simulink model "pid_extended_state_observor_pendulum"  (R2019b)
settings: Solver=FixedStepAuto  StartTime=0.0  StopTime=20  FixedStep=0.001  RelTol=1e-3
values from neighbouring files (symbols this model uses):
  L = [3*wd 3*wd^2 wd^3]'    [eso_design.m]
  wn = 1    [eso_design.m]
  zeta = 0.1    [eso_design.m]
libraries: simulink x1
settings Model: Creator=henry  LastModifiedBy=henry

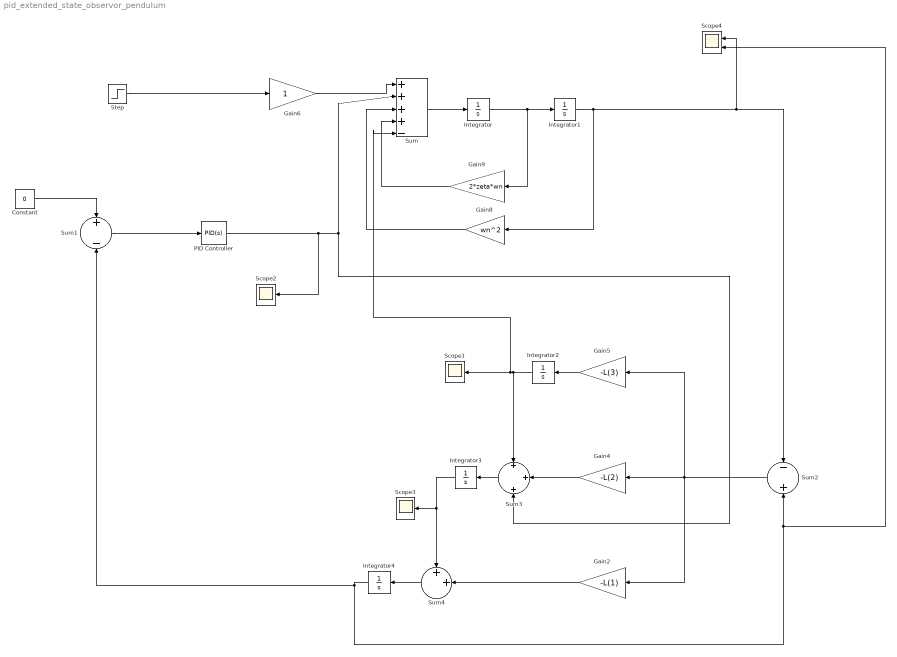
== system pid_extended_state_observor_pendulum ==
  Constant : Constant  Value=0
  Gain2 : Gain  Gain=-L(1)
  Gain4 : Gain  Gain=-L(2)
  Gain5 : Gain  Gain=-L(3)
  Gain6 : Gain
  Gain8 : Gain  Gain=wn^2
  Gain9 : Gain  Gain=2*zeta*wn
  Integrator : Integrator  InitialCondition=-1.5
  Integrator1 : Integrator  InitialCondition=0.5
  Integrator2 : Integrator
  Integrator3 : Integrator
  Integrator4 : Integrator
  PID Controller : simulink/Continuous/PID Controller  Controller=PID  Form=Ideal  TimeDomain=Continuous-time  SampleTime=-1  IntegratorMethod=Forward Euler  FilterMethod=Forward Euler  ControllerParametersSource=internal  P=10  I=5  D=1  UseFilter=on  N=100  TunerSelectOption=Transfer Function Based (PID Tuner App)  InitialConditionSource=internal  InitialConditionForIntegrator=0  InitialConditionForFilter=0  DifferentiatorICPrevScaledInput=0  ExternalReset=none  TrackingMode=off  Kt=1  LimitOutput=off  UpperSaturationLimit=inf  LowerSaturationLimit=-inf  LinearizeAsGain=on  AntiWindupMode=none  Kb=1  POutMin=[]  POutMax=[]  IOutMin=[]  IOutMax=[]  DOutMin=[]  DOutMax=[]  NOutMin=[]  NOutMax=[]  SumOutMin=[]  SumOutMax=[]  SaturationOutMin=[]  SaturationOutMax=[]  PParamMin=[]  PParamMax=[]  IParamMin=[]  IParamMax=[]  DParamMin=[]  DParamMax=[]  NParamMin=[]  NParamMax=[]  KbParamMin=[]  KbParamMax=[]  KtParamMin=[]  KtParamMax=[]  KbOutMin=[]  KbOutMax=[]  KtOutMin=[]  KtOutMax=[]  IntegratorOutMin=[]  IntegratorOutMax=[]  FilterOutMin=[]  FilterOutMax=[]  SumI1OutMin=[]  SumI1OutMax=[]  SumI2OutMin=[]  SumI2OutMax=[]  SumI3OutMin=[]  SumI3OutMax=[]  SumI4OutMin=[]  SumI4OutMax=[]  SumDOutMin=[]  SumDOutMax=[]  DifferentiatorOutMin=[]  DifferentiatorOutMax=[]  FilterDiffOutCoefMin=[]  FilterDiffOutCoefMax=[]  ReciprocalOutMin=[]  ReciprocalOutMax=[]  SumDenOutMin=[]  SumDenOutMax=[]  SumNumOutMin=[]  SumNumOutMax=[]  DivideOutMin=[]  DivideOutMax=[]  IntegratorContinuousStateAttributes=''  IntegratorStateMustResolveToSignalObject=off  IntegratorRTWStateStorageClass=Auto  FilterContinuousStateAttributes=''  FilterStateMustResolveToSignalObject=off  FilterRTWStateStorageClass=Auto  ParallelPVariant=Passthrough  IdealPVariant=InternalParameters  IVariant=InternalParameters  DVariant=InternalParameters  IntegratorVariant=Continuous  SatVariant=Disabled  AWVariant=Passthrough  PCopyVariant=Disabled  TRVariant=Disabled  FdbkBlocksVariant=Forward  IdealPFdbkVariant=Disabled  SatFdbkVariant=Disabled  DerivativeFilterVariant=ContFilter  NVariant=InternalParameters  NCopyVariant=Disabled  FilterICVariant=InternalICsFilter  IntegratorICVariant=InternalICs  ExternalResetVariant=Disabled  TRSumVariant=Passthrough  SumFdbkVariant=Disabled  SumVariant=Sum_PID
  Scope1 : Scope
  Scope2 : Scope
  Scope3 : Scope
  Scope4 : Scope  NumInputPorts=2
  Step : Step  Time=5  SampleTime=0
  Sum : Sum  Inputs=|++++-
  Sum1 : Sum  Inputs=+-
  Sum2 : Sum  Inputs=-|+
  Sum3 : Sum  Inputs=+|+|+
  Sum4 : Sum  Inputs=++|
  wires:
  Sum/1 -> Integrator/1
  Integrator/1 -> Integrator1/1, Gain9/1
  Sum2/1 -> Gain5/1, Gain2/1, Gain4/1
  Gain2/1 -> Sum4/2
  Gain4/1 -> Sum3/2
  Gain5/1 -> Integrator2/1
  Integrator2/1 -> Sum/5, Scope1/1, Sum3/1
  Sum3/1 -> Integrator3/1
  Integrator3/1 -> Scope3/1, Sum4/1
  Sum4/1 -> Integrator4/1
  Integrator4/1 -> Sum1/2, Scope4/2, Sum2/2
  Integrator1/1 -> Scope4/1, Sum2/1, Gain8/1
  Gain6/1 -> Sum/1
  Step/1 -> Gain6/1
  Gain8/1 -> Sum/3
  Gain9/1 -> Sum/4
  PID Controller/1 -> Scope2/1, Sum/2, Sum3/3
  Constant/1 -> Sum1/1
  Sum1/1 -> PID Controller/1
